simulink model "SFverinsA"  (R2020a)
settings: Solver=VariableStepAuto  StartTime=0.0  StopTime=inf  RelTol=1e-3
libraries: simulink x5
settings Model: Creator=maxen  LastModifiedBy=maxen

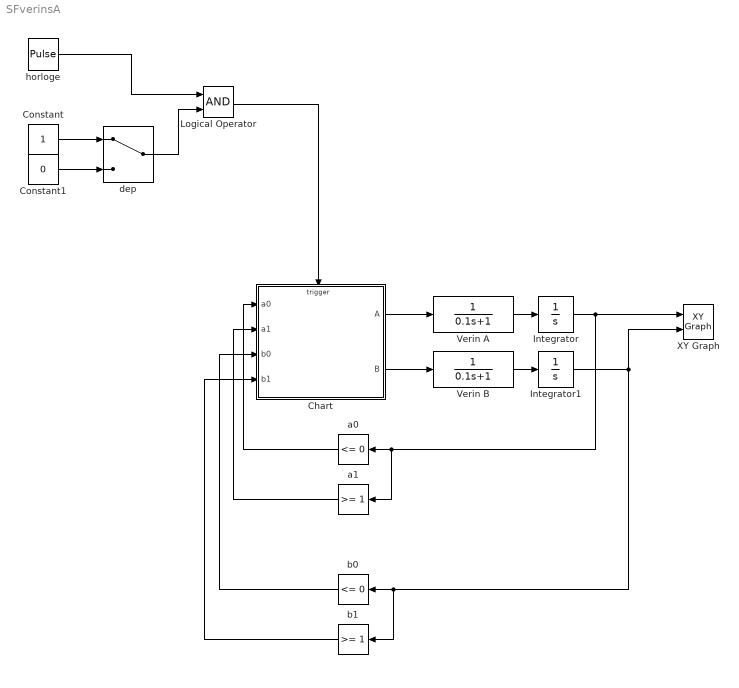
== system SFverinsA ==
  Chart : Stateflow chart  TreatAsAtomicUnit=on
  Constant : Constant
  Constant1 : Constant  Value=0
  Integrator : Integrator
  Integrator1 : Integrator
  Logical Operator : Logic  AllPortsSameDT=off  OutDataTypeStr=boolean
  Verin A : TransferFcn  Denominator=[0.1 1]
  Verin B : TransferFcn  Denominator=[0.1 1]
  XY Graph : simulink/Sinks/XY Graph  xmin=-2  xmax=2  ymin=-2  ymax=2  st=-1
  a0 : simulink/Logic and Bit Operations/Compare To Zero  relop=<=  OutDataTypeStr=boolean
  a1 : simulink/Logic and Bit Operations/Compare To Constant  relop=>=  const=1  OutDataTypeStr=boolean
  b0 : simulink/Logic and Bit Operations/Compare To Zero  relop=<=  OutDataTypeStr=boolean
  b1 : simulink/Logic and Bit Operations/Compare To Constant  relop=>=  const=1  OutDataTypeStr=boolean
  dep : ManualSwitch
  horloge : DiscretePulseGenerator  PulseType=Time based  Period=0.01  PulseWidth=5
  wires:
  Constant/1 -> dep/1
  Constant1/1 -> dep/2
  Chart/1(A) -> Verin A/1
  Chart/2(B) -> Verin B/1
  Verin A/1 -> Integrator/1
  Verin B/1 -> Integrator1/1
  Integrator/1 -> a1/1, a0/1, XY Graph/1
  Integrator1/1 -> XY Graph/2, b1/1, b0/1
  a0/1 -> Chart/1(a0)
  a1/1 -> Chart/2(a1)
  b0/1 -> Chart/3(b0)
  b1/1 -> Chart/4(b1)
  horloge/1 -> Logical Operator/1
  dep/1 -> Logical Operator/2
  Logical Operator/1 -> Chart/Trigger

== stateflow chart SFverinsA/Chart ==
  state No_A_B
    en:A=-1;
    en:B=-1;
  state Initial_State
    en:A=0;
    en:B=0;
  state Full_A_B
    en:A=0;
    en:B=1;
  state Full_A
    en:A=1;
  No_A_B -> Initial_State : [a0 && b0]
  (default) -> Initial_State
  Full_A_B -> No_A_B : [b1]
  Initial_State -> Full_A : [dep && a0 && b0]
  Full_A -> Full_A_B : [a1]
  data: a0 input; a1 input; b0 input; b1 input; A output; B output
  events: dep input EITHER_EDGE_EVENT
